simulink model "SegwayV1"  (R2021a)
settings: Solver=VariableStepAuto  StartTime=0.0  StopTime=10.0  RelTol=1e-3
values from neighbouring files (symbols this model uses):
  A = [0  1  0  0 ... (first row only)    [Segway_modelV1.m]    (also in Segway_modelV2.m)
  B = [0 ; B2 ; 0 ; B4;]    [Segway_modelV1.m]    (also in Segway_modelV2.m)
  C = [1 0 0 0 ... (first row only)    [Segway_modelV1.m]    (also in Segway_modelV2.m)
settings Model: Creator=mluser  LastModifiedBy=mluser

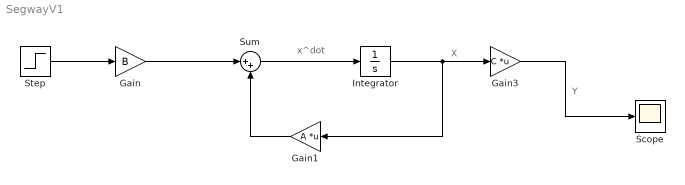
== system SegwayV1 ==
  note: Y
  note: X
  note: x^dot
  Gain : Gain  Gain=B
  Gain1 : Gain  Gain=A  Multiplication=Matrix(K*u)
  Gain3 : Gain  Gain=C  Multiplication=Matrix(K*u)
  Integrator : Integrator
  Scope : Scope
  Step : Step  SampleTime=0
  Sum : Sum  Inputs=|++
  wires:
  Sum/1 -> Integrator/1
  Gain/1 -> Sum/1
  Integrator/1 -> Gain1/1, Gain3/1
  Gain1/1 -> Sum/2
  Gain3/1 -> Scope/1
  Step/1 -> Gain/1
